simulink model "FluxWeakeningControl"  (R2026a)
settings: Solver=FixedStepDiscrete
undefined symbols (not defined in the file): flux_allowed_norm, flux_max, Id_Table, Iq_Table, torque_limit, trq_norm
libraries: sl_discontinuities x1
settings Model: DataDictionary=TractionEmotorSoftwareArchInterfaceData.sldd  Creator=dakaihu  LastModifiedBy=dakaihu
settings OptimizationCC: GainParamInheritBuiltInType=on  UseFloatMulNetSlope=on  InlineInvariantSignals=on  NoFixptDivByZeroProtection=on  EfficientFloat2IntCast=on  LifeSpan=1
settings HardwareCC: ProdBitPerChar=16.0  ProdBitPerInt=16.0  ProdLargestAtomicInteger=Integer  ProdWordSize=16.0  ProdHWDeviceType=Texas Instruments->C2000
settings RTWCC: SystemTargetFile=ert.tlc  GenCodeOnly=on  Description=Embedded Coder
settings CodeAppCC: MaxIdLength=40.0  CustomSymbolStrGlobalVar=rt$N$M  CustomSymbolStrType=$N$M  CustomSymbolStrFcn=$N$M$F  CustomSymbolStrMacro=$N$M  ReqsInCode=on
settings ERTTargetCC: ERTFilePackagingFormat=CompactWithDataFile  GenerateSampleERTMain=on  IncludeMdlTerminateFcn=off  CombineSignalStateStructs=on  SupportAbsoluteTime=off  SupportComplex=off

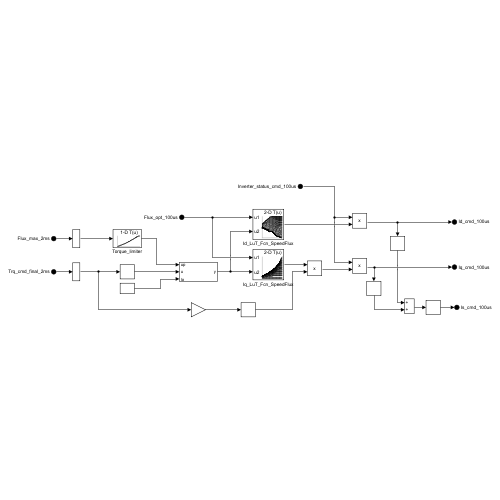
[thumbnail: Simulink's stored preview of the top-level diagram]
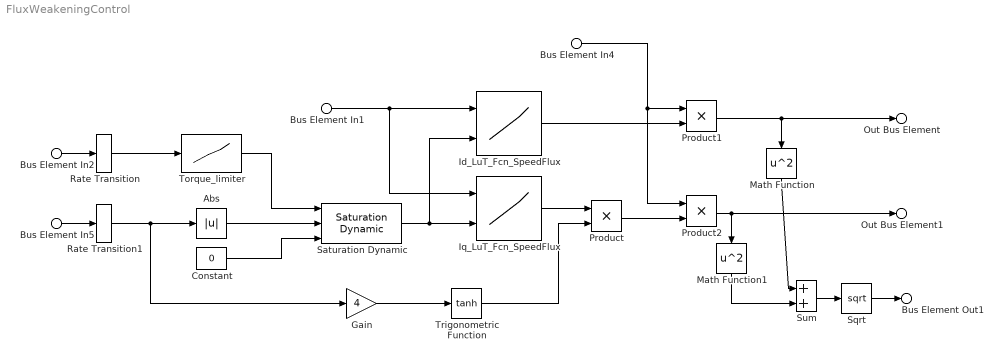
== system FluxWeakeningControl ==
  Bus Element In5 : Inport  PortName=Trq_cmd_final_2ms
  Bus Element In2 : Inport  Port=2  PortName=Flux_max_2ms
  Bus Element In4 : Inport  Port=3  PortName=Inverter_status_cmd_100us
  Bus Element In1 : Inport  Port=4  PortName=Flux_opt_100us
  Abs : Abs  SaturateOnIntegerOverflow=off
  Constant : Constant  Value=0  SampleTime=-1
  Gain : Gain  Gain=4
  Id_LuT_Fcn_SpeedFlux : Lookup_n-D  BreakpointsForDimension1=flux_allowed_norm  BreakpointsForDimension2=trq_norm  Table=Id_Table  ExtrapMethod=Clip  UseLastTableValue=on  InternalRulePriority=Speed  RndMeth=Simplest
      settings: InputPortMap=u0,u1
  Iq_LuT_Fcn_SpeedFlux : Lookup_n-D  BreakpointsForDimension1=flux_allowed_norm  BreakpointsForDimension2=trq_norm  Table=Iq_Table  ExtrapMethod=Clip  UseLastTableValue=on  InternalRulePriority=Speed  RndMeth=Simplest
      settings: InputPortMap=u0,u1
  Math Function : Math  Operator=square
  Math Function1 : Math  Operator=square
  Product : Product
  Product1 : Product
  Product2 : Product
  Rate Transition : RateTransition  Deterministic=off  OutPortSampleTime=1e-4
  Rate Transition1 : RateTransition  Deterministic=off  OutPortSampleTime=1e-4
  Saturation Dynamic : sl_discontinuities/Saturation Dynamic  OutMin=[]  OutMax=[]  OutDataTypeStr=Inherit: Same as second input  OutDataType=fixdt(1, 16)  OutScaling=2^-10  DoSatur=off
  Sqrt : Sqrt
  Sum : Sum
  Torque_limiter : Lookup_n-D  NumberOfTableDimensions=1  BreakpointsForDimension1=flux_max  Table=torque_limit  ExtrapMethod=Clip  UseLastTableValue=on  InternalRulePriority=Speed  RndMeth=Simplest
  Trigonometric Function : Trigonometry  Operator=tanh
  Bus Element Out1 : Outport  PortName=Is_cmd_100us
  Out Bus Element : Outport  Port=2  PortName=Id_cmd_100us
  Out Bus Element1 : Outport  Port=3  PortName=Iq_cmd_100us
  wires:
  Bus Element In2/1 -> Rate Transition/1
  Torque_limiter/1 -> Saturation Dynamic/1
  Constant/1 -> Saturation Dynamic/3
  Bus Element In5/1 -> Rate Transition1/1
  Abs/1 -> Saturation Dynamic/2
  Bus Element In1/1 -> Iq_LuT_Fcn_SpeedFlux/1, Id_LuT_Fcn_SpeedFlux/1
  Saturation Dynamic/1 -> Iq_LuT_Fcn_SpeedFlux/2, Id_LuT_Fcn_SpeedFlux/2
  Gain/1 -> Trigonometric Function/1
  Iq_LuT_Fcn_SpeedFlux/1 -> Product/1
  Trigonometric Function/1 -> Product/2
  Bus Element In4/1 -> Product2/1, Product1/1
  Product2/1 -> Math Function1/1, Out Bus Element1/1
  Product1/1 -> Out Bus Element/1, Math Function/1
  Id_LuT_Fcn_SpeedFlux/1 -> Product1/2
  Product/1 -> Product2/2
  Math Function/1 -> Sum/1
  Sum/1 -> Sqrt/1
  Math Function1/1 -> Sum/2
  Sqrt/1 -> Bus Element Out1/1
  Rate Transition/1 -> Torque_limiter/1
  Rate Transition1/1 -> Gain/1, Abs/1
